simulink model "ultracap_converter_simplified_PI_control_v5_mod_for_deployment"  (R2012b)
settings: Solver=ode45  StartTime=0.0  StopTime=4  FixedStep=TsampleSimulink  MaxStep=1e-6  RelTol=1e-3
values from neighbouring files (symbols this model uses):
  Ea = 4.2622    [me547_based_PI_controller_v3.m]
  Ra = 0.0560    (= 0.056)    [me547_based_PI_controller_v3.m]
  Ts = 1/fs    (= 0.0002)    [load_system_parameters.m]
  Vbat = 48    [load_system_parameters.m]
undefined symbols (not defined in the file or in its folder): DiscIntNeverNeededParam, ILcommand_z, plecs
libraries: simulink x1, dspsigops x1
settings Model: Creator=Raghav  LastModifiedBy=Raghav

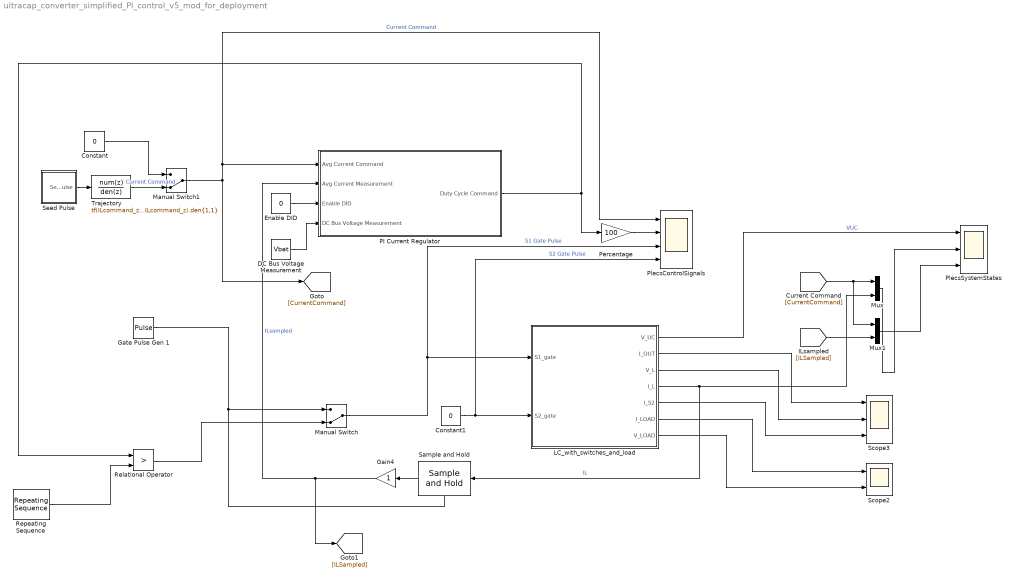
== system ultracap_converter_simplified_PI_control_v5_mod_for_deployment ==
  Constant : Constant  Value=0
  Constant1 : Constant  Value=0
  DC Bus Voltage Measurement : Constant  Value=Vbat
  Enable DID : Constant  Value=0
  Gain4 : Gain  SampleTime=Ts
  Gate Pulse Gen 1 : DiscretePulseGenerator  PulseType=Time based  Period=Ts  PulseWidth=71.42
  LC_with_switches_and_load : Subsystem  LoadFcn=plecs('sl', 200);  InitFcn=plecs('sl', 214);  StartFcn=plecs('sl', 208);  StopFcn=plecs('sl', 209);  mask(PlecsCircuit){PLECSData=<binary blob, 2116 chars, not shown>}
      mask prompts: PLECSData "PLECS Data (Do not delete or modify!)"
      mask init:
      | % PLACE CUSTOM INITIALIZATIONS ABOVE
      | % DO NOT REMOVE
      | plecs('sl', 215);
      | % DO NOT REMOVE
      settings: CopyFcn=plecs('sl', 203);  DeleteFcn=plecs('sl', 205);  UndoDeleteFcn=plecs('sl', 206);  PreSaveFcn=plecs('sl', 211);  PostSaveFcn=plecs('sl', 201);  NameChangeFcn=plecs('sl', 210);  DestroyFcn=plecs('sl', 207);  PreCopyFcn=plecs('sl', 216);  OpenFcn=plecs('sl', 202);  ErrorFcn=plerrorfcn
      mask Help: web(['file:///' fullfile(plecsdoc, 'creatingacircuit.html')])
      mask Display: disp('PLECS\nCircuit')
  Manual Switch : ManualSwitch  CurrentSetting=0
  Manual Switch1 : ManualSwitch  CurrentSetting=0
  Mux : Mux  Inputs=2
  Mux1 : Mux  Inputs=2
  PI Current Regulator : Subsystem
  Percentage : Gain  Gain=100
  PlecsControlSignals : Scope  NumInputPorts=4
      settings: YMin=0~0~-0.5~-0.5  YMax=5~1~1.5~1.5  SaveName=PlecsControlSignals
  PlecsSystemStates : Scope  NumInputPorts=3
      settings: ShowLegends=on  YMin=0~-50~-5  YMax=3.75~650~5  SaveName=PlecsSystemStates
  Relational Operator : RelationalOperator  Priority=50  Operator=>  OutDataTypeStr=boolean
  Repeating Sequence : simulink/Sources/Repeating Sequence  rep_seq_t=[0 Ts]  rep_seq_y=[0 1]
  Sample and Hold : dspsigops/Sample and Hold  trig=Rising edge  initCond=0  latchinput=on
  Scope2 : Scope  NumInputPorts=2
      settings: ShowLegends=on  YMin=-5~-5  YMax=5~5  SaveName=ScopeData2
  Scope3 : Scope  NumInputPorts=3
      settings: ShowLegends=on  YMin=0~-50~-5  YMax=3.75~650~5  SaveName=Scope3
  Seed Pulse : Subsystem
  Trajectory : DiscreteTransferFcn  Numerator=tf(ILcommand_z).num{1,1}  Denominator=tf(ILcommand_z).den{1,1}  SampleTime=Ts
  wires:
  LC_with_switches_and_load/1(V_UC) -> PlecsSystemStates/1  "VUC"
  LC_with_switches_and_load/7(V_LOAD) -> Scope2/2
  LC_with_switches_and_load/4(I_L) -> Mux/2, Sample and Hold/1  "IL"
  LC_with_switches_and_load/6(I_LOAD) -> Scope2/1
  Constant1/1 -> PlecsControlSignals/4, LC_with_switches_and_load/2(S2_gate)  "S2 Gate Pulse"
  Manual Switch/1 -> LC_with_switches_and_load/1(S1_gate), PlecsControlSignals/3  "S1 Gate Pulse"
  Seed Pulse/1(Seed Pulse) -> Trajectory/1
  Manual Switch1/1 -> PlecsControlSignals/1, PI Current Regulator/1(Avg Current Command), [CurrentCommand]  "Current Command"
  Repeating Sequence/1 -> Relational Operator/2
  Gate Pulse Gen 1/1 -> Sample and Hold/Trigger, Manual Switch/1
  Relational Operator/1 -> Manual Switch/2
  Sample and Hold/1 -> Gain4/1
  Gain4/1 -> PI Current Regulator/2(Avg Current Measurement), [ILSampled]  "ILsampled"
  LC_with_switches_and_load/2(I_OUT) -> Scope3/1
  LC_with_switches_and_load/3(V_L) -> Scope3/2
  LC_with_switches_and_load/5(I_S2) -> Scope3/3
  [CurrentCommand] -> Mux1/1, Mux/1
  Mux/1 -> PlecsSystemStates/2
  Mux1/1 -> PlecsSystemStates/3
  [ILSampled] -> Mux1/2
  Percentage/1 -> PlecsControlSignals/2
  Trajectory/1 -> Manual Switch1/2  "Current Command"
  Constant/1 -> Manual Switch1/1
  PI Current Regulator/1(Duty Cycle Command) -> Percentage/1, Relational Operator/1
  Enable DID/1 -> PI Current Regulator/3(Enable DID)
  DC Bus Voltage Measurement/1 -> PI Current Regulator/4(DC Bus Voltage Measurement)

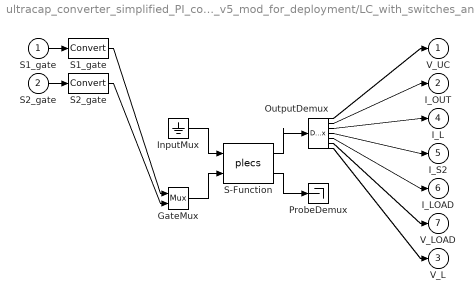
== system ultracap_converter_simplified_PI_control_v5_mod_for_deployment/LC_with_switches_and_load ==
  S1_gate : Inport  PortDimensions=1
  S2_gate : Inport  Port=2  PortDimensions=1
  " GateMux " : Mux  Inputs=[ 1 1 ]
  " InputMux " : Ground
  " OutputDemux " : Demux  Outputs=[ 1 1 1 1 1 1 1 ]
  " ProbeDemux " : Terminator
  " S-Function " : S-Function  FunctionName=plecs  EnableBusSupport=off
  " S1_gate " : DataTypeConversion  SaturateOnIntegerOverflow=on  RndMeth=Zero
  " S2_gate " : DataTypeConversion  SaturateOnIntegerOverflow=on  RndMeth=Zero
  V_UC : Outport  PortDimensions=1
  I_OUT : Outport  Port=2  PortDimensions=1
  V_L : Outport  Port=3  PortDimensions=1
  I_L : Outport  Port=4  PortDimensions=1
  I_S2 : Outport  Port=5  PortDimensions=1
  I_LOAD : Outport  Port=6  PortDimensions=1
  V_LOAD : Outport  Port=7  PortDimensions=1
  wires:
  " S-Function "/2 -> " ProbeDemux "/1
  " GateMux "/1 -> " S-Function "/2
  " InputMux "/1 -> " S-Function "/1
  " S-Function "/1 -> " OutputDemux "/1
  S1_gate/1 -> " S1_gate "/1
  " S1_gate "/1 -> " GateMux "/1
  S2_gate/1 -> " S2_gate "/1
  " S2_gate "/1 -> " GateMux "/2
  " OutputDemux "/1 -> V_UC/1
  " OutputDemux "/2 -> I_OUT/1
  " OutputDemux "/3 -> I_L/1
  " OutputDemux "/4 -> I_S2/1
  " OutputDemux "/5 -> I_LOAD/1
  " OutputDemux "/6 -> V_LOAD/1
  " OutputDemux "/7 -> V_L/1

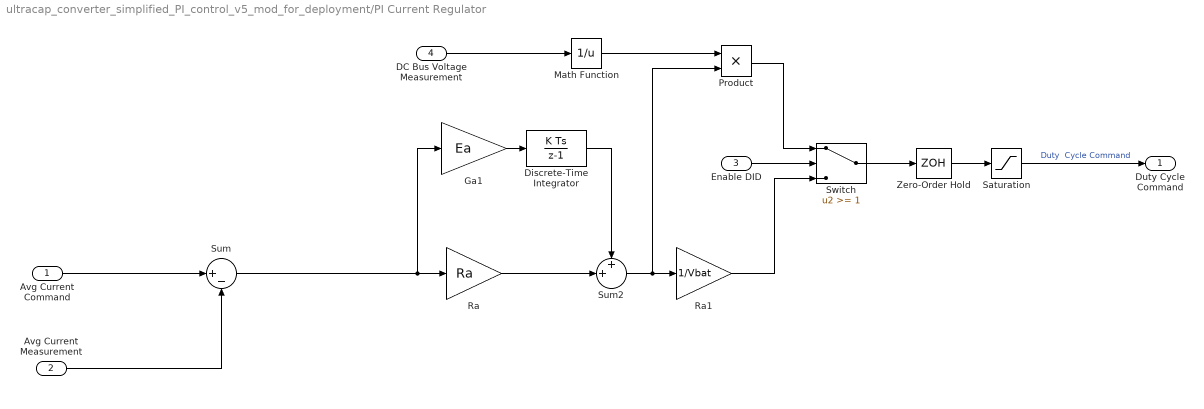
== system ultracap_converter_simplified_PI_control_v5_mod_for_deployment/PI Current Regulator ==
  Avg Current Command : Inport
  Avg Current Measurement : Inport  Port=2
  Enable DID : Inport  Port=3
  DC Bus Voltage Measurement : Inport  Port=4
  Discrete-Time Integrator : DiscreteIntegrator  SampleTime=Ts  LimitOutput=on  UpperSaturationLimit=5  LowerSaturationLimit=-5  ICPrevOutput=DiscIntNeverNeededParam  ICPrevScaledInput=DiscIntNeverNeededParam
  Ga1 : Gain  Gain=Ea  SampleTime=Ts
  Math Function : Math  Operator=reciprocal  SaturateOnIntegerOverflow=on
  Product : Product  RndMeth=Zero
  Ra : Gain  Gain=Ra  SampleTime=Ts
  Ra1 : Gain  Gain=1/Vbat  SampleTime=Ts
  Saturation : Saturate  UpperLimit=0.99  LowerLimit=0
  Sum : Sum  Inputs=|+-
  Sum2 : Sum  Inputs=++|
  Switch : Switch  Threshold=1
  Zero-Order Hold : ZeroOrderHold  SampleTime=Ts
  Duty Cycle Command : Outport
  wires:
  Ra1/1 -> Switch/3
  Sum/1 -> Ra/1, Ga1/1
  Saturation/1 -> Duty Cycle Command/1  "Duty  Cycle Command"
  Ga1/1 -> Discrete-Time Integrator/1
  Sum2/1 -> Product/2, Ra1/1
  Zero-Order Hold/1 -> Saturation/1
  Ra/1 -> Sum2/2
  Discrete-Time Integrator/1 -> Sum2/1
  Avg Current Measurement/1 -> Sum/2
  Avg Current Command/1 -> Sum/1
  Switch/1 -> Zero-Order Hold/1
  Enable DID/1 -> Switch/2
  DC Bus Voltage Measurement/1 -> Math Function/1
  Math Function/1 -> Product/1
  Product/1 -> Switch/1

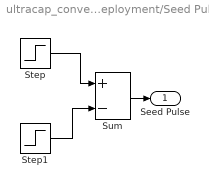
== system ultracap_converter_simplified_PI_control_v5_mod_for_deployment/Seed Pulse ==
  Step : Step  Time=10*Ts  SampleTime=0
  Step1 : Step  Time=10*Ts+Ts/2  SampleTime=0
  Sum : Sum  Inputs=+-
  Seed Pulse : Outport
  wires:
  Sum/1 -> Seed Pulse/1
  Step/1 -> Sum/1
  Step1/1 -> Sum/2
